simulink model "typeB"  (R2023b)
settings: Solver=VariableStepAuto  StartTime=0.0  StopTime=10.0  RelTol=1e-3
libraries: spsDCVoltageSourceLib x2, spsCurrentMeasurementLib x1, spsDiodeLib x1, spsIdealSwitchLib x1, spsSeriesRLCBranchLib x1, msbUtilities x1, spsVoltageMeasurementLib x1, sps_lib x1
settings Model: Creator=aryangoel  LastModifiedBy=aryangoel

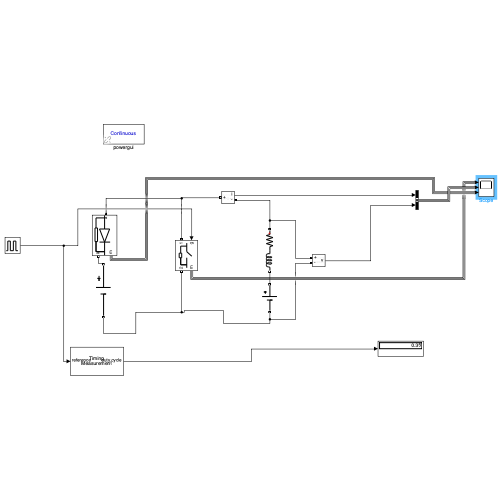
[thumbnail: Simulink's stored preview of the top-level diagram]
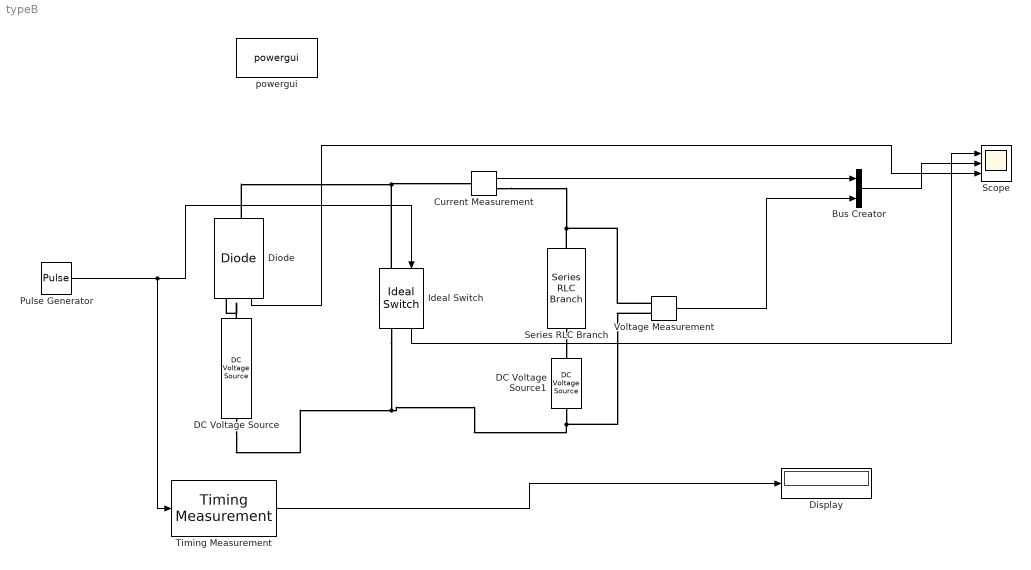
== system typeB ==
  Bus Creator : BusCreator  Inputs=2
  Current Measurement : spsCurrentMeasurementLib/Current Measurement  PhasorSimulation=off  OutputType=Complex  PSBequivalent=0
  DC Voltage Source : spsDCVoltageSourceLib/DC Voltage Source  Amplitude=120  Measurements=Voltage
  DC Voltage Source1 : spsDCVoltageSourceLib/DC Voltage Source  Amplitude=50  Measurements=Voltage
  Diode : spsDiodeLib/Diode  Ron=0.001  Lon=0  Vf=0.8  IC=0  UseSnubber=0  Rs=500  Cs=250e-9  Measurements=on
  Display : Display
      settings: Format=decimal (Stored Integer)
  Ideal Switch : spsIdealSwitchLib/Ideal Switch  Ron=0.001  Lon=0  IC=0  Rs=1e5  Cs=inf  Measurements=on
  Pulse Generator : DiscretePulseGenerator  PulseType=Time based  Period=1  PulseWidth=35
  Scope : Scope  NumInputPorts=3
  Series RLC Branch : spsSeriesRLCBranchLib/Series RLC Branch  LConnTagsString=__new0  RConnTagsString=__new0  BranchType=RL  Resistance=1000  Inductance=0.001  SetiL0=off  InitialCurrent=0  Capacitance=0  Setx0=off  InitialVoltage=0  Measurements=None
  Timing Measurement : msbUtilities/Timing Measurement  Period=off  Frequency=off  RiseTime=off  FallTime=off  DutyCycle=on  Delay=off  SameRefThreshold=on  GlobalRefThreshold=0  Range=[-1 1]  MeasurementType=80% / 20%  ThresholdMax=0.6  ThresholdMin=-0.6  DcRefThreshold=0  DelayRefThreshold=0  DelayTstThreshold=0
  Voltage Measurement : spsVoltageMeasurementLib/Voltage Measurement  PhasorSimulation=off  OutputType=Complex  PSBequivalent=0
  powergui : sps_lib/powergui  Priority=1  SimulationMode=Continuous  SampleTime=50e-6  frequency=60  Iterations=50  frequencyindice=0  Pbase=100e6  ErrMax=1e-4  UnitsV=kV  UnitsW=MW  buscounter=0  FunctionMessages=off  echomessages=off  EnableUseOfTLC=off  CurrentSourceSwitches=off  DisableSnubberDevices=off  DisableRonSwitches=off  DisableVfSwitches=off  DisplayEquations=off  AutomaticDiscreteSolvers=off  SolverType=Tustin/Backward Euler (TBE)  Interpol=off  ExternalGateDelay=off  methode=off  Ts=100  x0status=blocks  SPID=on  SwTol=0  HookPort=off  NonlinearTolerance=1e-4  nMaxIteration=100  ContinueOnMaxIteration=off  RestoreLinks=warning  ResistiveCurrentMeasurement=off  Frange=[0:2:500]  Ylog=off  Xlog=on  ShowGrid=off  save=off  variable=ZData  structure=0  ZoomFFT=off  StartTime=0.0  cycles=1  DisplayStyle=1  fundamental=60  FreqAxis=off  MaxFrequency=1000  frequencyindicesteady=1  RmsSteady=1  display=off
  wires:
  Pulse Generator/1 -> Timing Measurement/1, Ideal Switch/1
  Current Measurement/1 -> Bus Creator/1
  Diode/1 -> Scope/3
  Voltage Measurement/1 -> Bus Creator/2
  Timing Measurement/1 -> Display/1
  Ideal Switch/1 -> Scope/1
  Bus Creator/1 -> Scope/2
  connections:
  DC Voltage Source/LConn1 -- Ideal Switch/RConn1 -- Voltage Measurement/LConn2 -- DC Voltage Source1/LConn1
  Current Measurement/RConn1 -- Series RLC Branch/LConn1 -- Voltage Measurement/LConn1
  Ideal Switch/LConn1 -- Diode/LConn1 -- Current Measurement/LConn1
  DC Voltage Source/RConn1 -- Diode/RConn1
  Series RLC Branch/RConn1 -- DC Voltage Source1/RConn1
